simulink model "sensor"  (R2018b)
settings: Solver=VariableStepAuto  StartTime=0.0  StopTime=Endtime  RelTol=1e-3
values from neighbouring files (symbols this model uses):
  alpha_T = 1.5/1000    (= 0.0015)    [plant_model_sim.m]    (also in sensor_sim.m)
  omega_d = 2*pi    (= 6.28318530718)    [plant_model_sim.m]    (also in sensor_sim.m)
libraries: simulink x1
settings Model: Creator=nharada  LastModifiedBy=nharada

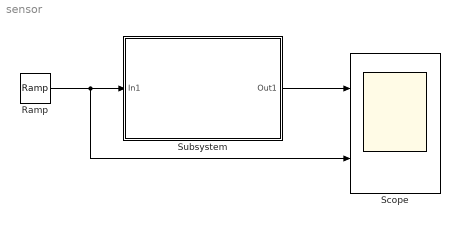
== system sensor ==
  Ramp : simulink/Sources/Ramp  slope=omega_d  start=10  InitialOutput=0
  Scope : Scope  NumInputPorts=2
  Subsystem : Subsystem
  wires:
  Ramp/1 -> Scope/2, Subsystem/1(In1)
  Subsystem/1(Out1) -> Scope/1

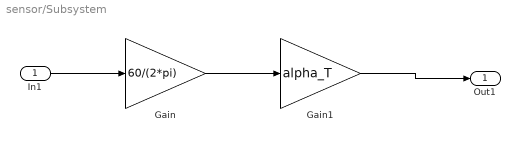
== system sensor/Subsystem ==
  In1 : Inport
  Gain : Gain  Gain=60/(2*pi)
  Gain1 : Gain  Gain=alpha_T
  Out1 : Outport
  wires:
  In1/1 -> Gain/1
  Gain/1 -> Gain1/1
  Gain1/1 -> Out1/1
